simulink model "arduinoTemplate"  (R2018a)
settings: Solver=FixedStepAuto  StartTime=0.0  StopTime=inf  RelTol=1e-3  EnableMultiTasking=on
PreLoadFcn:
  | addpath(genpath('Drivers'))
libraries: arduinoDrivers_lib x9
settings Model: SimulationMode=external  ExtModeTrigDuration=2  Creator=Raphael  LastModifiedBy=Raphael
settings OptimizationCC: MaxStackSize=64
settings DebuggingCC: ParameterTunabilityLossMsg=error
settings HardwareCC: ProdBitPerInt=16  ProdBitPerPointer=16  ProdBitPerSizeT=16  ProdBitPerPtrDiffT=16  ProdLargestAtomicFloat=None  ProdWordSize=8  ProdHWDeviceType=Atmel->AVR
settings SFSimCC: MATLABDynamicMemAlloc=off
settings RTWCC: SystemTargetFile=ert.tlc  HardwareBoard=Arduino Mega 2560  TLCOptions=-aInlineSetEventsForThisBaseRateFcn=TLC_FALSE -aSuppressMultiTaskScheduler=TLC_FALSE -aRateBasedStepFcn=1  TemplateMakefile=ert_default_tmf  GenerateReport=on  Toolchain=Arduino AVR  BuildConfiguration=Faster Runs  IncludeHyperlinkInReport=on  GenerateTraceInfo=on  GenerateTraceReport=on  GenerateTraceReportSl=on  GenerateTraceReportSf=on  GenerateTraceReportEml=on
settings CodeAppCC: ForceParamTrailComments=on  IgnoreCustomStorageClasses=off  OperatorAnnotations=on  SimulinkDataObjDesc=on  SFDataObjDesc=on  MATLABFcnDesc=on  InsertBlockDesc=on  StateflowObjectComments=on  MATLABSourceComments=on
settings ERTTargetCC: MultiwordLength=2048  SupportContinuousTime=on  SupportVariableSizeSignals=on

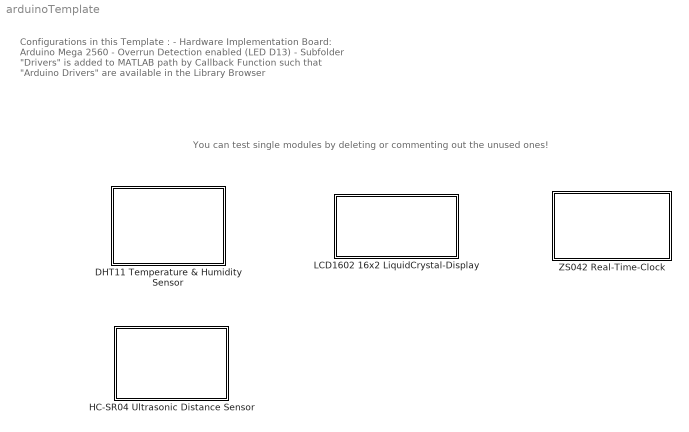
== system arduinoTemplate ==
  note: You can test single modules by deleting or commenting out the unused ones!
  note: Configurations in this Template :
      |
      | - Hardware Implementation Board: Arduino Mega 2560
      | - Overrun Detection enabled (LED D13)
      | - Subfolder "Drivers" is added to MATLAB path by Callback Function
      | such that "Arduino Drivers" are available in the Library Browser
  DHT11 Temperature & Humidity Sensor : Subsystem
      mask Display: image('DHT11.jpg');
  HC-SR04 Ultrasonic Distance Sensor : Subsystem
      mask Display: image('HC-SR04.jpg');
  LCD1602 16x2 LiquidCrystal-Display : Subsystem
      mask Display: image('LCD1602.jpg');
  ZS042 Real-Time-Clock : Subsystem
      mask Display: image('ZS-042.png');

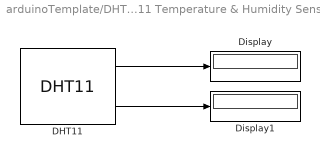
== system arduinoTemplate/DHT11 Temperature & Humidity Sensor ==
  DHT11 : arduinoDrivers_lib/DHT11 Temperature & Humidity Sensor/DHT11  pin_Mask=44  tS_Mask=1
      settings: SourceProductName=Arduino Drivers
  Display : Display
  Display1 : Display
  wires:
  DHT11/1 -> Display/1
  DHT11/2 -> Display1/1

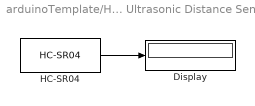
== system arduinoTemplate/HC-SR04 Ultrasonic Distance Sensor ==
  Display : Display
  HC-SR04 : arduinoDrivers_lib/HC-SR04 Ultrasonic Distance Sensor/HC-SR04  trig_Mask=7  echo_Mask=6  tS_Mask=1
      settings: SourceProductName=Arduino Drivers
  wires:
  HC-SR04/1 -> Display/1

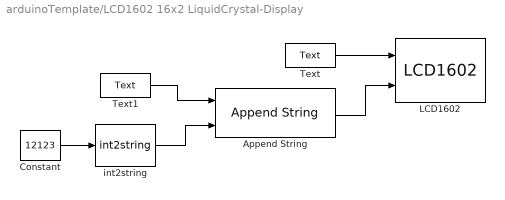
== system arduinoTemplate/LCD1602 16x2 LiquidCrystal-Display ==
  Append String : arduinoDrivers_lib/LCD1602 16x2 LiquidCrystal-Display/Append String
      settings: SourceProductName=Arduino Drivers
  Constant : Constant  Value=12123
  LCD1602 : arduinoDrivers_lib/LCD1602 16x2 LiquidCrystal-Display/LCD1602  rs_Mask=26  en_Mask=27  d4_Mask=22  d5_Mask=23  d6_Mask=24  d7_Mask=25
      settings: SourceProductName=Arduino Drivers
  Text : arduinoDrivers_lib/LCD1602 16x2 LiquidCrystal-Display/Text  text_Mask='ExampleText'  SampleTime=inf
      settings: SourceProductName=Arduino Drivers
  Text1 : arduinoDrivers_lib/LCD1602 16x2 LiquidCrystal-Display/Text  text_Mask='Test-No.: '  SampleTime=inf
      settings: SourceProductName=Arduino Drivers
  int2string : arduinoDrivers_lib/LCD1602 16x2 LiquidCrystal-Display/int2string
      settings: SourceProductName=Arduino Drivers
  wires:
  Text1/1 -> Append String/1
  Text/1 -> LCD1602/1
  int2string/1 -> Append String/2
  Append String/1 -> LCD1602/2
  Constant/1 -> int2string/1

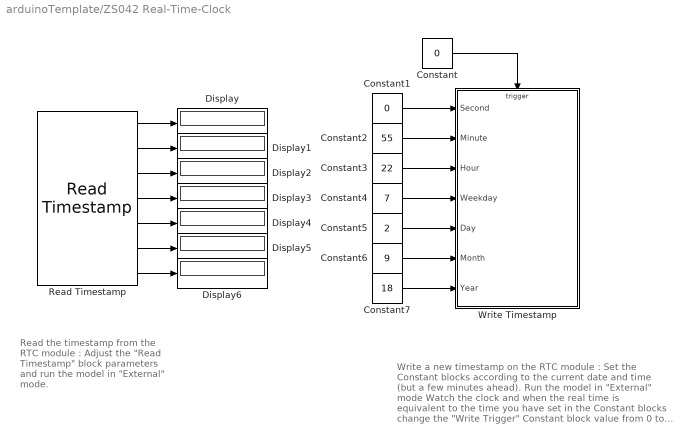
== system arduinoTemplate/ZS042 Real-Time-Clock ==
  note: Write a new timestamp on the RTC module :
      |
      | Set the Constant blocks according to the current date and time (but a few minutes ahead).
      | Run the model in "External" mode
      | Watch the clock and when the real time is equivalent to the time you have set in the Constant blocks change the "Write Trigger" Constant block value from 0 to 1 suddenly.
  note: Read the timestamp from the RTC module :
      |
      | Adjust the "Read Timestamp" block parameters and run the model in "External" mode.
  Constant : Constant  Value=0
  Constant1 : Constant  Value=0
  Constant2 : Constant  Value=55
  Constant3 : Constant  Value=22
  Constant4 : Constant  Value=7
  Constant5 : Constant  Value=2
  Constant6 : Constant  Value=9
  Constant7 : Constant  Value=18
  Display{,1..6} (7 alike) : Display
  Read Timestamp : arduinoDrivers_lib/ZS042 Real-Time-Clock/Read Timestamp  tsMask=1
      settings: SourceProductName=Arduino Drivers
  Write Timestamp : Subsystem
  wires:
  Read Timestamp/3 -> Display2/1
  Read Timestamp/4 -> Display3/1
  Read Timestamp/2 -> Display1/1
  Read Timestamp/1 -> Display/1
  Read Timestamp/5 -> Display4/1
  Read Timestamp/6 -> Display5/1
  Read Timestamp/7 -> Display6/1
  Constant/1 -> Write Timestamp/Trigger
  Constant1/1 -> Write Timestamp/1(Second)
  Constant2/1 -> Write Timestamp/2(Minute)
  Constant3/1 -> Write Timestamp/3(Hour)
  Constant4/1 -> Write Timestamp/4(Weekday)
  Constant5/1 -> Write Timestamp/5(Day)
  Constant6/1 -> Write Timestamp/6(Month)
  Constant7/1 -> Write Timestamp/7(Year)

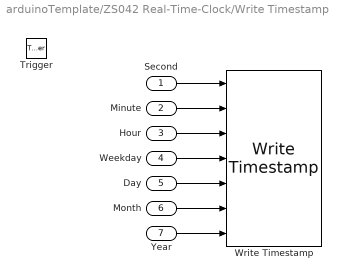
== system arduinoTemplate/ZS042 Real-Time-Clock/Write Timestamp ==
  Second : Inport
  Minute : Inport  Port=2
  Hour : Inport  Port=3
  Weekday : Inport  Port=4
  Day : Inport  Port=5
  Month : Inport  Port=6
  Year : Inport  Port=7
  Trigger : TriggerPort  VariantControl=Variant  PortDimensions=1
  Write Timestamp : arduinoDrivers_lib/ZS042 Real-Time-Clock/Write Timestamp
      settings: SourceProductName=Arduino Drivers
  wires:
  Second/1 -> Write Timestamp/1
  Minute/1 -> Write Timestamp/2
  Hour/1 -> Write Timestamp/3
  Weekday/1 -> Write Timestamp/4
  Day/1 -> Write Timestamp/5
  Month/1 -> Write Timestamp/6
  Year/1 -> Write Timestamp/7
